simulink model "CCL_1"  (R2018a)
settings: Solver=ode4  StartTime=0  StopTime=inf  MaxStep=1e-4  RelTol=1e-3
InitFcn:
  | close
  | clear
  | clc
  | Sc=128
  | f=60;
  | T=1/f;
  | Ts=1/(f*Sc);
  | Vr=6500
  | V_v=[1    0.4    1          0.6       1       0.6       1       0.75   0.95]
  | T_v=[0   20/f  70/f    200/f   300/f     330/f   400/f   500/f  10]
  | S_time=60/f*20.5
  | V_R=3;
  | Tf=3
  | T_lc=3
  | set_param('CCL_1/EMISOR-RECEPTOR/TCP_IP_RX/ESCRITURA','Value','[0,0,0]')
undefined symbols (not defined in the file or in its folder): man, Vuc
libraries: libreria_comunicaciones_servidor1 x2, powerlib x1
settings Model: Creator=Mateo  LastModifiedBy=ana-n
settings CodeAppCC: StateflowObjectComments=on
settings SimscapeCC: SimscapeNormalizeSystem=off

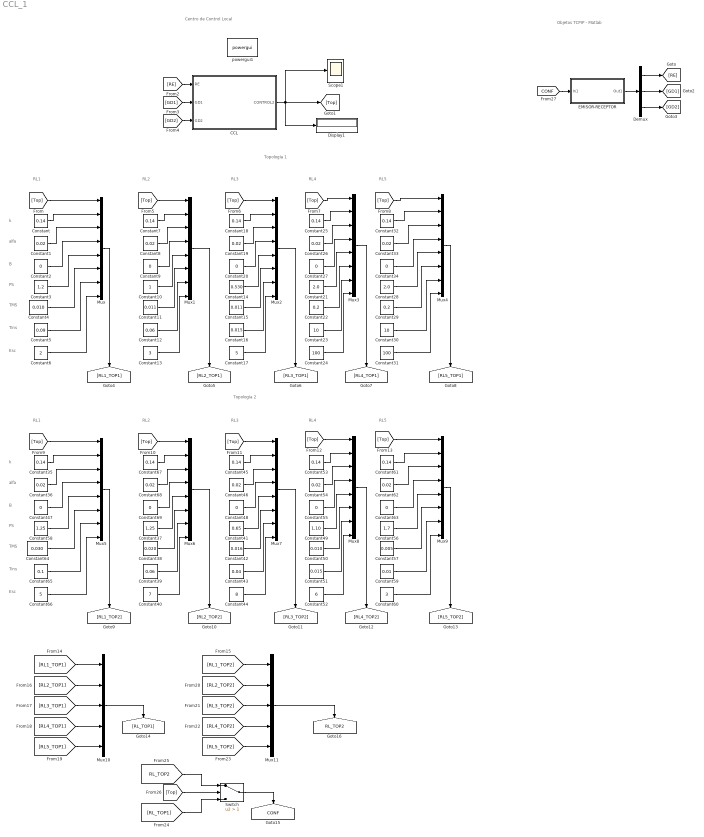
== system CCL_1 ==
  note: k
  note: Centro de Control Local
  note: Objetos TCPIP - Matlab
  note: alfa
  note: B
  note: PS
  note: TMS
  note: Tins
  note: Esc
  note: RL1
  note: RL2
  note: RL3
  note: RL4
  note: RL5
  note: Topología 1
  note: Topología 2
  note: k
  note: alfa
  note: B
  note: PS
  note: TMS
  note: Tins
  note: Esc
  note: RL1
  note: RL2
  note: RL3
  note: RL4
  note: RL5
  CCL : Subsystem  mask(Selector de topología de operación del sistema IEEE de 34 barras){modo=Automática, manual=Con GD}
      mask help: Bloque del centro de control local con configuración manual y automática.
      mask TypeOptions modo: Automática | Manual
      mask Callback modo:
      | h1 = getSimulinkBlockHandle(gcb);
      | modo = get_param(h1,'modo');
      | if strcmp(modo,'Automática')
      |     Vuc=1;
      |     set_param(h1,'MaskVisibilities',{'on','off'});
      |     man=0;
      | elseif strcmp(modo,'Manual')
      |     Vuc=0;
      |     set_param(h1,'MaskVisibilities',{'on','on'});
      | end
      mask TypeOptions manual: Radial | Con GD
      mask Callback manual:
      | clc,
      | h2 = getSimulinkBlockHandle(gcb);
      | manuales = get_param(h2,'manual');
      | if strcmp(manuales,'Radial')
      |     man=1;
      | elseif strcmp(manuales,'Con GD')
      |     man=2;
      | end
      mask DialogControl ParameterGroupVar Prompt: Selección del tipo de configuración del sistema IEEE de 34 barras
      mask Display:
      | color('black');
      | disp('CCL');
      | port_label('input',1,'RE');
      | port_label('input',2,'GD1');
      | port_label('input',3,'GD2');
      | port_label('output',1,'Param');
  Constant{,7,18,25,32,35,45,53,61,67} (10 alike) : Constant  Value=0.14
  Constant{1,8,19,26,33,36,46,54,62,68} (10 alike) : Constant  Value=0.02
  Constant10 : Constant
  Constant11 : Constant  Value=0.011
  Constant12 : Constant  Value=0.06
  Constant13 : Constant  Value=3
  Constant14 : Constant  Value=0.530
  Constant15 : Constant  Value=0.011
  Constant16 : Constant  Value=0.015
  Constant17 : Constant  Value=5
  Constant{2,9,20,27,34,47..48,55,63,69} (10 alike) : Constant  Value=0
  Constant21 : Constant  Value=2.0
  Constant22 : Constant  Value=0.2
  Constant23 : Constant  Value=10
  Constant24 : Constant  Value=100
  Constant28 : Constant  Value=2.0
  Constant29 : Constant  Value=0.2
  Constant3 : Constant  Value=1.2
  Constant30 : Constant  Value=10
  Constant31 : Constant  Value=100
  Constant37 : Constant  Value=1.25
  Constant38 : Constant  Value=0.020
  Constant39 : Constant  Value=0.06
  Constant4 : Constant  Value=0.010
  Constant40 : Constant  Value=7
  Constant41 : Constant  Value=0.65
  Constant42 : Constant  Value=0.016
  Constant43 : Constant  Value=0.04
  Constant44 : Constant  Value=8
  Constant49 : Constant  Value=1.10
  Constant5 : Constant  Value=0.09
  Constant50 : Constant  Value=0.010
  Constant51 : Constant  Value=0.015
  Constant52 : Constant  Value=6
  Constant56 : Constant  Value=1.7
  Constant57 : Constant  Value=0.005
  Constant58 : Constant  Value=1.25
  Constant59 : Constant  Value=0.01
  Constant6 : Constant  Value=2
  Constant60 : Constant  Value=3
  Constant64 : Constant  Value=0.030
  Constant65 : Constant  Value=0.1
  Constant66 : Constant  Value=5
  Demux : Demux  Outputs=3
  Display1 : Display
  EMISOR-RECEPTOR : Subsystem
      mask Display:
      | color('black');
      | port_label('input',1,'Emisor');
      | port_label('output',1,'Receptor');
  Mux{,1..9} (10 alike) : Mux  Inputs=8
  Mux10 : Mux  Inputs=5
  Mux11 : Mux  Inputs=5
  Scope1 : Scope
  Switch : Switch  Criteria=u2 > Threshold  Threshold=1
  powergui1 : powerlib/powergui  Priority=1  SimulationMode=Discrete  SampleTime=1/(60*256)  frequency=60  Iterations=50  frequencyindice=0  Pbase=100e6  ErrMax=1e-4  UnitsV=kV  UnitsW=MW  buscounter=0  FunctionMessages=off  echomessages=off  EnableUseOfTLC=off  CurrentSourceSwitches=on  DisableSnubberDevices=off  DisableRonSwitches=off  DisableVfSwitches=off  DisplayEquations=off  SolverType=Tustin/Backward Euler (TBE)  Interpol=off  ExternalGateDelay=off  methode=off  Ts=10  x0status=blocks  SPID=off  SwTol=0  HookPort=off  RestoreLinks=warning  ResistiveCurrentMeasurement=off  Frange=[0:2:500]  Ylog=off  Xlog=on  ShowGrid=off  save=off  variable=ZData  structure=0  ZoomFFT=off  StartTime=0.0  cycles=1  DisplayStyle=1  fundamental=60  FreqAxis=off  MaxFrequency=1000  frequencyindicesteady=1  RmsSteady=1  display=off
  tag scope: CONF=global, RL_TOP2=global
  wires:
  CCL/1(CONTROL2) -> Scope1/1, Display1/1, [Top]
  Demux/1 -> [RE]
  Demux/2 -> [GD1]
  Demux/3 -> [GD2]
  [GD1] -> CCL/2(GD1)
  [RE] -> CCL/1(RE)
  [GD2] -> CCL/3(GD2)
  [Top] -> Mux/1
  Constant/1 -> Mux/2
  Constant1/1 -> Mux/3
  Constant2/1 -> Mux/4
  Constant3/1 -> Mux/5
  Constant4/1 -> Mux/6
  Constant5/1 -> Mux/7
  Constant6/1 -> Mux/8
  [Top] -> Mux1/1
  Constant7/1 -> Mux1/2
  Constant8/1 -> Mux1/3
  Constant9/1 -> Mux1/4
  Constant10/1 -> Mux1/5
  Constant11/1 -> Mux1/6
  Constant12/1 -> Mux1/7
  Constant13/1 -> Mux1/8
  [Top] -> Mux2/1
  Constant18/1 -> Mux2/2
  Constant19/1 -> Mux2/3
  Constant20/1 -> Mux2/4
  Constant14/1 -> Mux2/5
  Constant15/1 -> Mux2/6
  Constant16/1 -> Mux2/7
  Constant17/1 -> Mux2/8
  [Top] -> Mux3/1
  Constant25/1 -> Mux3/2
  Constant26/1 -> Mux3/3
  Constant27/1 -> Mux3/4
  Constant21/1 -> Mux3/5
  Constant22/1 -> Mux3/6
  Constant23/1 -> Mux3/7
  Constant24/1 -> Mux3/8
  [Top] -> Mux4/1
  Constant32/1 -> Mux4/2
  Constant33/1 -> Mux4/3
  Constant34/1 -> Mux4/4
  Constant28/1 -> Mux4/5
  Constant29/1 -> Mux4/6
  Constant30/1 -> Mux4/7
  Constant31/1 -> Mux4/8
  Mux/1 -> [RL1_TOP1]
  Mux1/1 -> [RL2_TOP1]
  Mux2/1 -> [RL3_TOP1]
  Mux3/1 -> [RL4_TOP1]
  Mux4/1 -> [RL5_TOP1]
  Mux9/1 -> [RL5_TOP2]
  Mux8/1 -> [RL4_TOP2]
  Mux7/1 -> [RL3_TOP2]
  Mux6/1 -> [RL2_TOP2]
  Mux5/1 -> [RL1_TOP2]
  Constant60/1 -> Mux9/8
  Constant59/1 -> Mux9/7
  Constant57/1 -> Mux9/6
  Constant56/1 -> Mux9/5
  Constant63/1 -> Mux9/4
  Constant62/1 -> Mux9/3
  Constant61/1 -> Mux9/2
  [Top] -> Mux9/1
  Constant52/1 -> Mux8/8
  Constant51/1 -> Mux8/7
  Constant50/1 -> Mux8/6
  Constant49/1 -> Mux8/5
  Constant55/1 -> Mux8/4
  Constant54/1 -> Mux8/3
  Constant53/1 -> Mux8/2
  [Top] -> Mux8/1
  Constant44/1 -> Mux7/8
  Constant43/1 -> Mux7/7
  Constant42/1 -> Mux7/6
  Constant41/1 -> Mux7/5
  Constant48/1 -> Mux7/4
  Constant46/1 -> Mux7/3
  Constant45/1 -> Mux7/2
  [Top] -> Mux7/1
  Constant40/1 -> Mux6/8
  Constant39/1 -> Mux6/7
  Constant38/1 -> Mux6/6
  Constant37/1 -> Mux6/5
  Constant69/1 -> Mux6/4
  Constant68/1 -> Mux6/3
  Constant67/1 -> Mux6/2
  [Top] -> Mux6/1
  Constant66/1 -> Mux5/8
  Constant65/1 -> Mux5/7
  Constant64/1 -> Mux5/6
  Constant58/1 -> Mux5/5
  Constant47/1 -> Mux5/4
  Constant36/1 -> Mux5/3
  Constant35/1 -> Mux5/2
  [Top] -> Mux5/1
  [RL1_TOP1] -> Mux10/1
  [RL2_TOP1] -> Mux10/2
  [RL3_TOP1] -> Mux10/3
  [RL4_TOP1] -> Mux10/4
  [RL5_TOP1] -> Mux10/5
  [RL5_TOP2] -> Mux11/5
  [RL4_TOP2] -> Mux11/4
  [RL3_TOP2] -> Mux11/3
  [RL2_TOP2] -> Mux11/2
  [RL1_TOP2] -> Mux11/1
  Mux10/1 -> [RL_TOP1]
  Mux11/1 -> [RL_TOP2]
  [Top] -> Switch/2
  [RL_TOP2] -> Switch/1
  [RL_TOP1] -> Switch/3
  Switch/1 -> [CONF]
  [CONF] -> EMISOR-RECEPTOR/1(In1)
  EMISOR-RECEPTOR/1(Out1) -> Demux/1

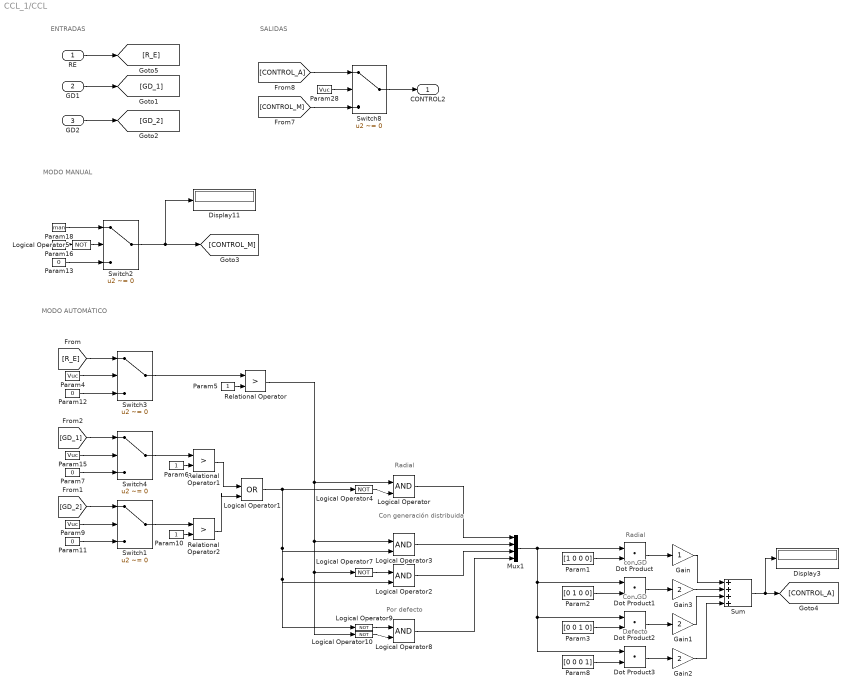
== system CCL_1/CCL ==
  note: MODO MANUAL
  note: MODO AUTOMÁTICO
  note: SALIDAS
  note: ENTRADAS
  note: con GD
  note: Por defecto
  note: Radial
  note: Radial
  note: Defecto
  note: Con generación
      | distribuida
  note: Con GD
  RE : Inport
  GD1 : Inport  Port=2
  GD2 : Inport  Port=3
  Display11 : Display
  Display3 : Display
  Dot Product{,1..3} (4 alike) : DotProduct  InputSameDT=on  OutDataTypeStr=Inherit: Inherit via internal rule
  Gain : Gain
  Gain1 : Gain  Gain=2
  Gain2 : Gain  Gain=2
  Gain3 : Gain  Gain=2
  Logical Operator{,2..3,8} (4 alike) : Logic  IconShape=distinctive  AllPortsSameDT=off  OutDataTypeStr=boolean
  Logical Operator1 : Logic  Operator=OR  IconShape=distinctive  AllPortsSameDT=off  OutDataTypeStr=boolean
  Logical Operator{4..5,7,9..10} (5 alike) : Logic  Operator=NOT  AllPortsSameDT=off  OutDataTypeStr=boolean
  Mux1 : Mux
  Param1 : Constant  Value=[1 0 0 0]  OutDataTypeStr=boolean
  Param10 : Constant
  Param{7,11..13} (4 alike) : Constant  Value=0
  Param{4,9,15..16,28} (5 alike) : Constant  Value=Vuc
  Param18 : Constant  Value=man
  Param2 : Constant  Value=[0 1 0 0]  OutDataTypeStr=boolean
  Param3 : Constant  Value=[0 0 1 0]  OutDataTypeStr=boolean
  Param5 : Constant
  Param6 : Constant
  Param8 : Constant  Value=[0 0 0 1]  OutDataTypeStr=boolean
  Relational Operator : RelationalOperator  Operator=>  OutDataTypeStr=boolean  RndMeth=Nearest
  Relational Operator1 : RelationalOperator  Operator=>  OutDataTypeStr=boolean  RndMeth=Nearest
  Relational Operator2 : RelationalOperator  Operator=>  OutDataTypeStr=boolean  RndMeth=Nearest
  Sum : Sum  Inputs=+|+|+|+
  Switch{1..4,8} (5 alike) : Switch  Criteria=u2 ~= 0
  CONTROL2 : Outport
  wires:
  RE/1 -> [R_E]
  Switch8/1 -> CONTROL2/1
  Param28/1 -> Switch8/2
  [CONTROL_M] -> Switch8/3
  [CONTROL_A] -> Switch8/1
  Switch2/1 -> Display11/1, [CONTROL_M]
  Param16/1 -> Logical Operator5/1
  Param13/1 -> Switch2/3
  Param18/1 -> Switch2/1
  Logical Operator5/1 -> Switch2/2
  GD1/1 -> [GD_1]
  GD2/1 -> [GD_2]
  Logical Operator4/1 -> Logical Operator/2
  Param6/1 -> Relational Operator1/2
  Switch3/1 -> Relational Operator/1
  Param5/1 -> Relational Operator/2
  Gain2/1 -> Sum/4
  Logical Operator/1 -> Mux1/1
  Switch4/1 -> Relational Operator1/1
  Param1/1 -> Dot Product/2
  Mux1/1 -> Dot Product3/1, Dot Product2/1, Dot Product1/1, Dot Product/1
  Dot Product/1 -> Gain/1
  Logical Operator8/1 -> Mux1/4
  Logical Operator10/1 -> Logical Operator8/2
  Relational Operator/1 -> Logical Operator7/1, Logical Operator10/1, Logical Operator3/1, Logical Operator/1
  Param15/1 -> Switch4/2
  Param4/1 -> Switch3/2
  Param12/1 -> Switch3/3
  Gain3/1 -> Sum/2
  Dot Product3/1 -> Gain2/1
  Param3/1 -> Dot Product2/2
  [R_E] -> Switch3/1
  Logical Operator9/1 -> Logical Operator8/1
  [GD_1] -> Switch4/1
  Gain/1 -> Sum/1
  Param2/1 -> Dot Product1/2
  Param8/1 -> Dot Product3/2
  Dot Product2/1 -> Gain1/1
  Sum/1 -> [CONTROL_A], Display3/1
  Dot Product1/1 -> Gain3/1
  Param7/1 -> Switch4/3
  Gain1/1 -> Sum/3
  Param11/1 -> Switch1/3
  [GD_2] -> Switch1/1
  Param9/1 -> Switch1/2
  Switch1/1 -> Relational Operator2/1
  Param10/1 -> Relational Operator2/2
  Relational Operator1/1 -> Logical Operator1/1
  Relational Operator2/1 -> Logical Operator1/2
  Logical Operator1/1 -> Logical Operator9/1, Logical Operator2/2, Logical Operator3/2, Logical Operator4/1
  Logical Operator7/1 -> Logical Operator2/1
  Logical Operator3/1 -> Mux1/2
  Logical Operator2/1 -> Mux1/3

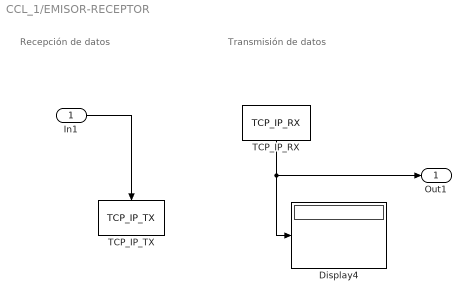
== system CCL_1/EMISOR-RECEPTOR ==
  note: Recepción de datos
  note: Transmisión de datos
  In1 : Inport
  Display4 : Display
  TCP_IP_RX : libreria_comunicaciones_servidor1/TCP_IP_RX  SystemSampleTime=-1
      link override ESCRITURA: Value=server_1.dato_lectura
  TCP_IP_TX : libreria_comunicaciones_servidor1/TCP_IP_TX  SystemSampleTime=-1
  Out1 : Outport
  wires:
  TCP_IP_RX/1 -> Out1/1, Display4/1
  In1/1 -> TCP_IP_TX/1
